simulink model "relay_2_vi_tri_r2015a"  (R2016b)
settings: Solver=ode4  StartTime=0.0  StopTime=30  FixedStep=1e-5  RelTol=1e-3
settings Model: Creator=ryell  LastModifiedBy=ADMIN
settings OptimizationCC: LifeSpan=inf
settings DebuggingCC: SFExecutionAtInitializationDiag=none
settings HardwareCC: ProdBitPerSizeT=32  ProdBitPerPtrDiffT=32  ProdWordSize=32  ProdHWDeviceType=Specified

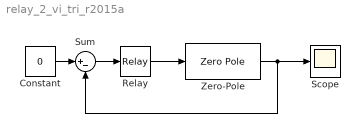
== system relay_2_vi_tri_r2015a ==
  Constant : Constant  Value=0
  Relay : Relay  OnOutputValue=4  OffOutputValue=-4
  Scope : Scope
  Sum : Sum  Inputs=|+-
  Zero-Pole : ZeroPole  Zeros=[]  Poles=[0 -1 -1]
  wires:
  Zero-Pole/1 -> Scope/1, Sum/2
  Constant/1 -> Sum/1
  Sum/1 -> Relay/1
  Relay/1 -> Zero-Pole/1
